simulink model "Part1"  (R2024b)
settings: Solver=VariableStepAuto  StartTime=0.0  StopTime=150  RelTol=1e-10
settings Model: Creator=baley  LastModifiedBy=baley
settings SolverCC: MaxConsecutiveMinStep=100

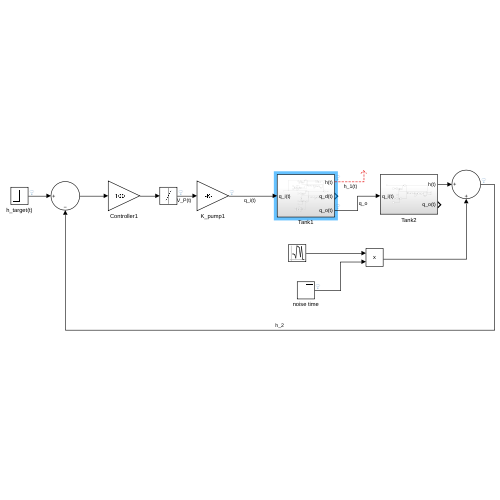
[thumbnail: Simulink's stored preview of the top-level diagram]
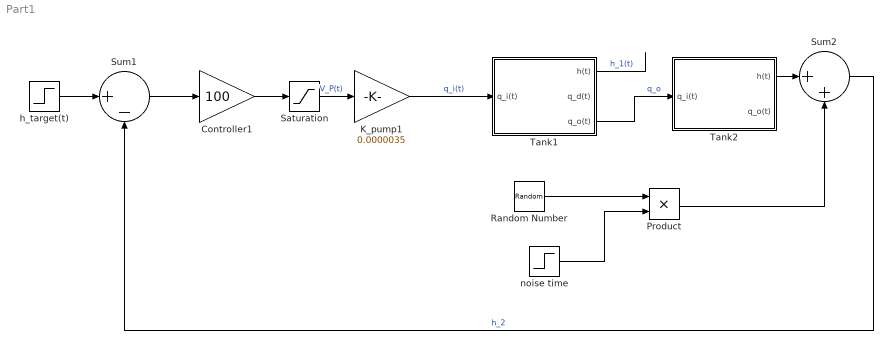
== system Part1 ==
  Controller1 : Gain  Gain=100
  K_pump1 : Gain  Gain=0.0000035
  Product : Product
  Random Number : RandomNumber  Variance=1e-6  SampleTime=0.1
  Saturation : Saturate  UpperLimit=12  LowerLimit=0
  Sum1 : Sum  Inputs=|+-
  Sum2 : Sum  Inputs=|++
  Tank1 : Subsystem
  Tank2 : Subsystem
  h_target(t) : Step  Before=10e-3  After=11e-3  SampleTime=0
  noise time : Step  Time=100  SampleTime=0
  wires:
  Sum1/1 -> Controller1/1
  h_target(t)/1 -> Sum1/1
  K_pump1/1 -> Tank1/1(q_i(t))  "q_i(t)"
  Controller1/1 -> Saturation/1
  Saturation/1 -> K_pump1/1  "V_P(t)"
  Tank2/1(h(t)) -> Sum2/1
  Sum2/1 -> Sum1/2  "h_2"
  Random Number/1 -> Product/1
  noise time/1 -> Product/2
  Product/1 -> Sum2/2
  Tank1/3(q_o(t)) -> Tank2/1(q_i(t))  "q_o"
  Tank1/1(h(t)) -> ?  "h_1(t)"

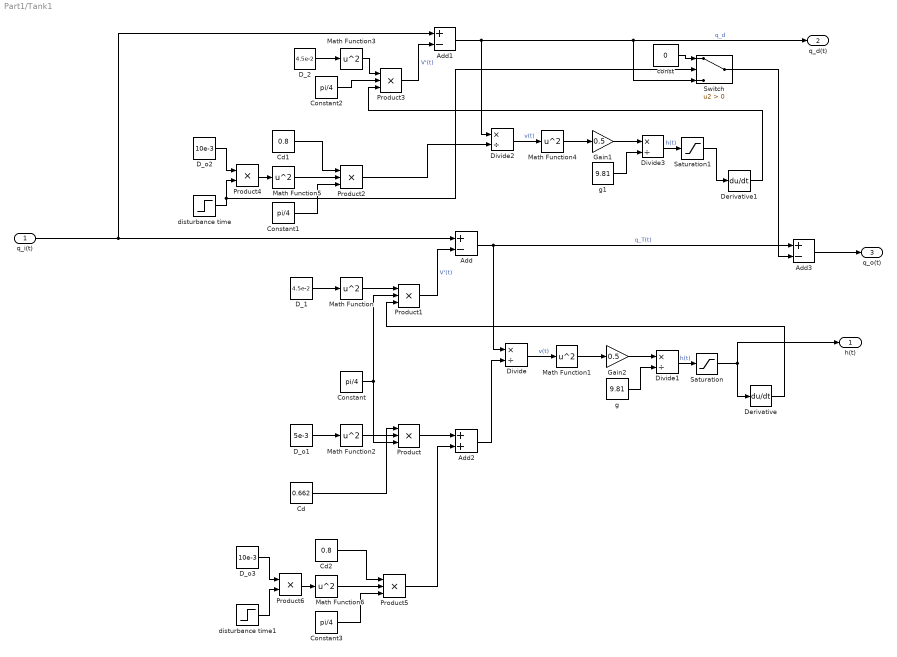
== system Part1/Tank1 ==
  q_i(t) : Inport
  Add : Sum  Inputs=+-
  Add1 : Sum  Inputs=+-
  Add2 : Sum
  Add3 : Sum  Inputs=+-
  Cd : Constant  Value=0.662
  Cd1 : Constant  Value=0.8
  Cd2 : Constant  Value=0.8
  Constant{,1..3} (4 alike) : Constant  Value=pi/4
  D_1 : Constant  Value=4.5e-2
  D_2 : Constant  Value=4.5e-2
  D_o1 : Constant  Value=5e-3
  D_o2 : Constant  Value=10e-3
  D_o3 : Constant  Value=10e-3
  Derivative : Derivative
  Derivative1 : Derivative
  Divide{,1..3} (4 alike) : Product  Inputs=*/
  Gain1 : Gain  Gain=0.5
  Gain2 : Gain  Gain=0.5
  Math Function{,1..6} (7 alike) : Math  Operator=square
  Product{,1..3,5} (5 alike) : Product  Inputs=3
  Product4 : Product
  Product6 : Product
  Saturation : Saturate  UpperLimit=25e-3  LowerLimit=0
  Saturation1 : Saturate  UpperLimit=25e-3  LowerLimit=0
  Switch : Switch  Criteria=u2 > Threshold  SaturateOnIntegerOverflow=off  InputSameDT=off
  const : Constant  Value=0
  disturbance time : Step  Time=45  Before=1e-100  SampleTime=0
  disturbance time1 : Step  Time=45  SampleTime=0
  g : Constant  Value=9.81
  g1 : Constant  Value=9.81
  h(t) : Outport
  q_d(t) : Outport  Port=2
  q_o(t) : Outport  Port=3
  wires:
  Cd/1 -> Product/1
  Constant/1 -> Product/3, Product1/2
  D_1/1 -> Math Function/1
  g/1 -> Divide1/2
  Math Function1/1 -> Gain2/1
  D_o1/1 -> Math Function2/1
  Add/1 -> Add3/1, Divide/1  "q_T(t)"
  Math Function2/1 -> Product/2
  Math Function/1 -> Product1/1
  Divide1/1 -> Saturation/1  "h(t)"
  Product1/1 -> Add/2  "V'(t)"
  Gain2/1 -> Divide1/1
  Divide/1 -> Math Function1/1  "v(t)"
  Derivative/1 -> Product1/3
  Saturation/1 -> h(t)/1, Derivative/1
  Constant1/1 -> Product2/3
  Add1/1 -> Divide2/1, Switch/3, q_d(t)/1  "q_d"
  Cd1/1 -> Product2/1
  q_i(t)/1 -> Add1/1, Add/1
  Math Function5/1 -> Product2/2
  D_o2/1 -> Product4/1
  Product4/1 -> Math Function5/1
  disturbance time/1 -> Switch/2, Product4/2
  Math Function3/1 -> Product3/1
  Product3/1 -> Add1/2  "V'(t)"
  Constant2/1 -> Product3/2
  D_2/1 -> Math Function3/1
  Divide3/1 -> Saturation1/1  "h(t)"
  Math Function4/1 -> Gain1/1
  Gain1/1 -> Divide3/1
  Divide2/1 -> Math Function4/1  "v(t)"
  Derivative1/1 -> Product3/3
  Saturation1/1 -> Derivative1/1
  g1/1 -> Divide3/2
  Product2/1 -> Divide2/2
  disturbance time1/1 -> Product6/2
  D_o3/1 -> Product6/1
  Math Function6/1 -> Product5/2
  Product6/1 -> Math Function6/1
  Constant3/1 -> Product5/3
  Cd2/1 -> Product5/1
  Product5/1 -> Add2/2
  Product/1 -> Add2/1
  Add2/1 -> Divide/2
  Add3/1 -> q_o(t)/1
  Switch/1 -> Add3/2
  const/1 -> Switch/1

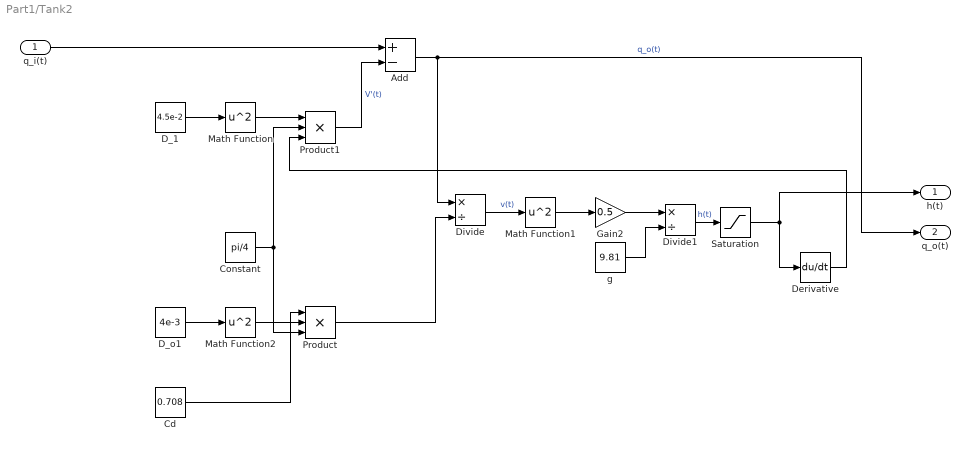
== system Part1/Tank2 ==
  q_i(t) : Inport
  Add : Sum  Inputs=+-
  Cd : Constant  Value=0.708
  Constant : Constant  Value=pi/4
  D_1 : Constant  Value=4.5e-2
  D_o1 : Constant  Value=4e-3
  Derivative : Derivative
  Divide : Product  Inputs=*/
  Divide1 : Product  Inputs=*/
  Gain2 : Gain  Gain=0.5
  Math Function : Math  Operator=square
  Math Function1 : Math  Operator=square
  Math Function2 : Math  Operator=square
  Product : Product  Inputs=3
  Product1 : Product  Inputs=3
  Saturation : Saturate  UpperLimit=25e-3  LowerLimit=0
  g : Constant  Value=9.81
  h(t) : Outport
  q_o(t) : Outport  Port=2
  wires:
  Cd/1 -> Product/1
  Constant/1 -> Product/3, Product1/2
  D_1/1 -> Math Function/1
  g/1 -> Divide1/2
  Math Function1/1 -> Gain2/1
  D_o1/1 -> Math Function2/1
  Add/1 -> q_o(t)/1, Divide/1  "q_o(t)"
  Math Function2/1 -> Product/2
  Math Function/1 -> Product1/1
  q_i(t)/1 -> Add/1
  Divide1/1 -> Saturation/1  "h(t)"
  Product/1 -> Divide/2
  Product1/1 -> Add/2  "V'(t)"
  Gain2/1 -> Divide1/1
  Divide/1 -> Math Function1/1  "v(t)"
  Derivative/1 -> Product1/3
  Saturation/1 -> Derivative/1, h(t)/1
